simulink model "Model_03_SS_RRF_PMSM_Model"  (R2020a)
settings: Solver=ode4  StartTime=0.0  StopTime=2  FixedStep=1e-4  RelTol=1e-3
settings Model: Creator=samee  LastModifiedBy=DEVIKAT
settings DebuggingCC: UnconnectedInputMsg=none  UnconnectedOutputMsg=none  UnconnectedLineMsg=none

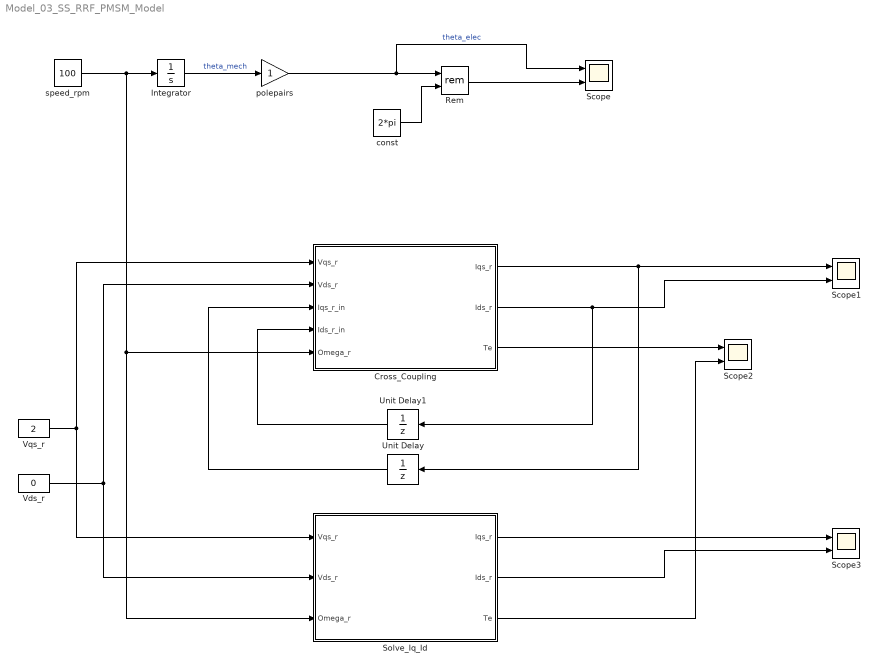
== system Model_03_SS_RRF_PMSM_Model ==
  Cross_Coupling : MATLAB Function  TreatAsAtomicUnit=on
  Integrator : Integrator
  Rem : Math  Operator=rem  SaturateOnIntegerOverflow=on
  Scope{,1..3} (4 alike) : Scope  NumInputPorts=2
  Solve_Iq_Id : MATLAB Function  TreatAsAtomicUnit=on
  Unit Delay : UnitDelay  SampleTime=-1  HasFrameUpgradeWarning=on
  Unit Delay1 : UnitDelay  SampleTime=-1  HasFrameUpgradeWarning=on
  Vds_r : Constant  Value=0
  Vqs_r : Constant  Value=2
  const : Constant  Value=2*pi
  polepairs : Gain
  speed_rpm : Constant  Value=100
  wires:
  Integrator/1 -> polepairs/1  "theta_mech"
  polepairs/1 -> Scope/1, Rem/1  "theta_elec"
  const/1 -> Rem/2
  Rem/1 -> Scope/2
  speed_rpm/1 -> Solve_Iq_Id/3(Omega_r), Cross_Coupling/5(Omega_r), Integrator/1
  Cross_Coupling/1(Iqs_r) -> Unit Delay/1, Scope1/1
  Cross_Coupling/2(Ids_r) -> Unit Delay1/1, Scope1/2
  Cross_Coupling/3(Te) -> Scope2/1
  Solve_Iq_Id/1(Iqs_r) -> Scope3/1
  Solve_Iq_Id/2(Ids_r) -> Scope3/2
  Vqs_r/1 -> Solve_Iq_Id/1(Vqs_r), Cross_Coupling/1(Vqs_r)
  Vds_r/1 -> Solve_Iq_Id/2(Vds_r), Cross_Coupling/2(Vds_r)
  Unit Delay/1 -> Cross_Coupling/3(Iqs_r_in)
  Unit Delay1/1 -> Cross_Coupling/4(Ids_r_in)
  Solve_Iq_Id/3(Te) -> Scope2/2

== matlab function Model_03_SS_RRF_PMSM_Model/Solve_Iq_Id ==
  data: Iqs_r output; Vqs_r input; Ids_r output; Te output; Vds_r input; Omega_r input
function [Iqs_r, Ids_r, Te] = fcn(Vqs_r, Vds_r, Omega_r)

rs          = 0.2;          %Stator resistance
Lq          = 300e-6;       %d and q axis inductances
Ld          = 300e-6;
Lambda_m_r  = 0.01;         %rotor flux linkages (back-emf constant)
P           = 2;            %number of poles


% Iqs_r = (1/rs)*(Vqs_r - Omega_r*Lambda_m_r - Omega_r*Ld*Ids_r_in); 
% Ids_r = (1/rs)*(Vds_r + Omega_r*Lq*Iqs_r_in);


K1 = ((rs^2)+(Omega_r^2)*Ld*Lq);

% Motor currents in rotor reference frame
Iqs_r = (rs/K1)*(Vqs_r - Omega_r*Lambda_m_r - (Omega_r*Ld/rs) *Vds_r); 
Ids_r = (1/K1)*(rs*Vds_r + Omega_r*Lq*Vqs_r - (Omega_r^2)*Lq*Lambda_m_r);

% Electromagnetic torque generated
Te = (3/2)*(P/2)*(Lambda_m_r*Iqs_r +(Ld-Lq)*Iqs_r*Ids_r);

== matlab function Model_03_SS_RRF_PMSM_Model/Cross_Coupling ==
  data: Iqs_r output; Vqs_r input; Ids_r output; Te output; Vds_r input; Iqs_r_in input; Ids_r_in input; Omega_r input
function [Iqs_r,Ids_r,Te] = fcn(Vqs_r,Vds_r,Iqs_r_in,Ids_r_in,Omega_r)

rs          = 0.2;      %Stator resistance
Lq          = 300e-6;   %d and q axis inductances
Ld          = 300e-6;
Lambda_m_r  = 0.01;     %rotor flux linkages (back-emf constant)
P           = 2;        %poles


Iqs_r = (1/rs)*(Vqs_r - Omega_r*Lambda_m_r - Omega_r*Ld*Ids_r_in);
Ids_r = (1/rs)*(Vds_r + Omega_r*Lq*Iqs_r_in); % using old Iq value which is 1 sample earlier

Te = (3/2)*(P/2)*(Lambda_m_r*Iqs_r + (Ld-Lq)*Iqs_r*Ids_r);
